simulink model "diff_derive"  (R2019b)
settings: Solver=VariableStepAuto  StartTime=0.0  StopTime=20  RelTol=1e-3
undefined symbols (not defined in the file): d1, DiscIntNeverNeededParam, Goal, p1, p2
libraries: simulink x2
settings Model: Creator=alilf  LastModifiedBy=alilf

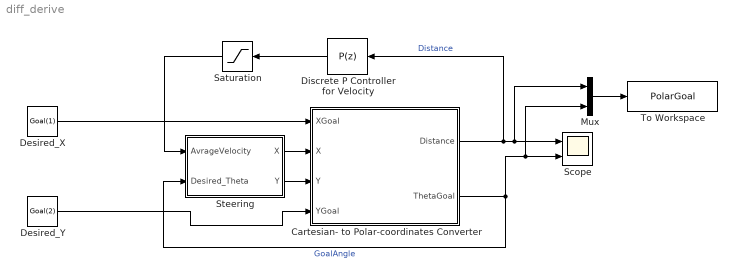
== system diff_derive ==
  "Cartesian- to Polar-coordinates Converter " : MATLAB Function  TreatAsAtomicUnit=on
  Desired_X : Constant  Value=Goal(1)  SampleTime=0.1
  Desired_Y : Constant  Value=Goal(2)  SampleTime=0.1
  Discrete P Controller for Velocity : simulink/Continuous/PID Controller  Controller=P  Form=Parallel  TimeDomain=Discrete-time  SampleTime=0.1  IntegratorMethod=Forward Euler  FilterMethod=Forward Euler  ControllerParametersSource=internal  P=p2  I=1  D=0  UseFilter=on  N=100  TunerSelectOption=Transfer Function Based (PID Tuner App)  InitialConditionSource=internal  InitialConditionForIntegrator=0  InitialConditionForFilter=0  DifferentiatorICPrevScaledInput=0  ExternalReset=none  TrackingMode=off  Kt=1  LimitOutput=off  UpperSaturationLimit=inf  LowerSaturationLimit=-inf  LinearizeAsGain=off  AntiWindupMode=none  Kb=1  POutMin=[]  POutMax=[]  IOutMin=[]  IOutMax=[]  DOutMin=[]  DOutMax=[]  NOutMin=[]  NOutMax=[]  SumOutMin=[]  SumOutMax=[]  SaturationOutMin=[]  SaturationOutMax=[]  PParamMin=[]  PParamMax=[]  IParamMin=[]  IParamMax=[]  DParamMin=[]  DParamMax=[]  NParamMin=[]  NParamMax=[]  KbParamMin=[]  KbParamMax=[]  KtParamMin=[]  KtParamMax=[]  KbOutMin=[]  KbOutMax=[]  KtOutMin=[]  KtOutMax=[]  IntegratorOutMin=[]  IntegratorOutMax=[]  FilterOutMin=[]  FilterOutMax=[]  SumI1OutMin=[]  SumI1OutMax=[]  SumI2OutMin=[]  SumI2OutMax=[]  SumI3OutMin=[]  SumI3OutMax=[]  SumI4OutMin=[]  SumI4OutMax=[]  SumDOutMin=[]  SumDOutMax=[]  DifferentiatorOutMin=[]  DifferentiatorOutMax=[]  FilterDiffOutCoefMin=[]  FilterDiffOutCoefMax=[]  ReciprocalOutMin=[]  ReciprocalOutMax=[]  SumDenOutMin=[]  SumDenOutMax=[]  SumNumOutMin=[]  SumNumOutMax=[]  DivideOutMin=[]  DivideOutMax=[]  IntegratorContinuousStateAttributes=''  IntegratorStateMustResolveToSignalObject=off  IntegratorRTWStateStorageClass=Auto  FilterContinuousStateAttributes=''  FilterStateMustResolveToSignalObject=off  FilterRTWStateStorageClass=Auto  ParallelPVariant=InternalParameters  IdealPVariant=Disabled  IVariant=Disabled  DVariant=Disabled  IntegratorVariant=Disabled  SatVariant=Disabled  AWVariant=Disabled  PCopyVariant=Disabled  TRVariant=Disabled  FdbkBlocksVariant=Forward  IdealPFdbkVariant=Disabled  SatFdbkVariant=Disabled  DerivativeFilterVariant=Disabled  NVariant=Disabled  NCopyVariant=Disabled_SignalSpec  FilterICVariant=Disabled  IntegratorICVariant=Disabled  ExternalResetVariant=Disabled  TRSumVariant=Passthrough  SumFdbkVariant=Disabled  SumVariant=Passthrough_P
  Mux : Mux  Inputs=2
  Saturation : Saturate  UpperLimit=8  LowerLimit=-8
  Scope : Scope  NumInputPorts=2
  "Steering " : Subsystem
  To Workspace : ToWorkspace  VariableName=PolarGoal  SaveFormat=Timeseries  SampleTime=-1
  wires:
  Saturation/1 -> "Steering "/1(AvrageVelocity)
  "Cartesian- to Polar-coordinates Converter "/2(ThetaGoal) -> Mux/2, Scope/2, "Steering "/2(Desired_Theta)  "GoalAngle"
  Discrete P Controller for Velocity/1 -> Saturation/1
  "Cartesian- to Polar-coordinates Converter "/1(Distance) -> Mux/1, Scope/1, Discrete P Controller for Velocity/1  "Distance"
  "Steering "/1(X) -> "Cartesian- to Polar-coordinates Converter "/2(X)
  "Steering "/2(Y) -> "Cartesian- to Polar-coordinates Converter "/3(Y)
  Desired_X/1 -> "Cartesian- to Polar-coordinates Converter "/1(XGoal)
  Desired_Y/1 -> "Cartesian- to Polar-coordinates Converter "/4(YGoal)
  Mux/1 -> To Workspace/1

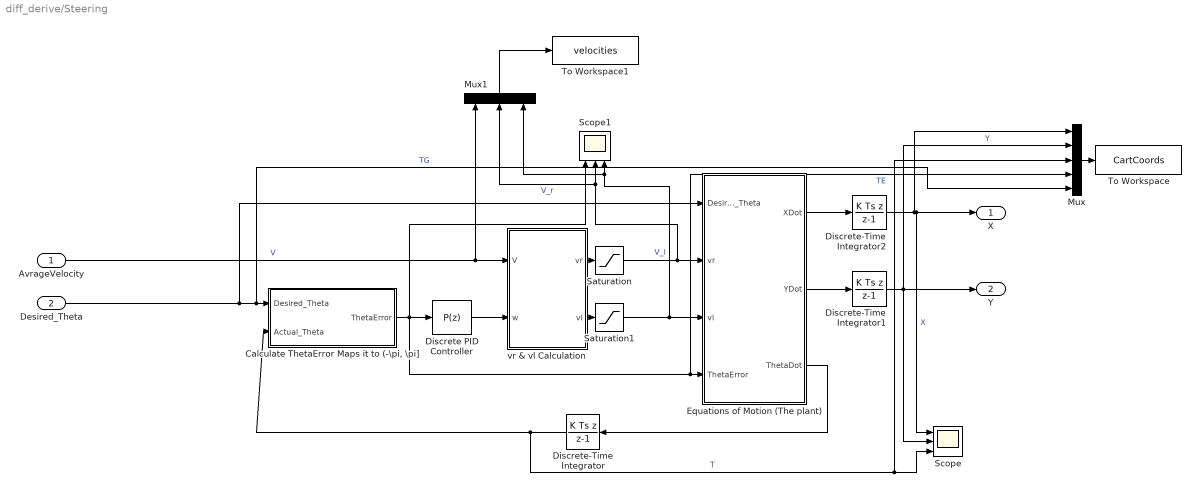
== system diff_derive/Steering  ==
  AvrageVelocity : Inport
  Desired_Theta : Inport  Port=2
  "Calculate ThetaError Maps it to (-\\pi, \\pi]" : MATLAB Function  TreatAsAtomicUnit=on
  Discrete PID Controller : simulink/Continuous/PID Controller  Controller=P  Form=Parallel  TimeDomain=Discrete-time  SampleTime=0.1  IntegratorMethod=Forward Euler  FilterMethod=Forward Euler  ControllerParametersSource=internal  P=p1  I=1  D=d1  UseFilter=on  N=100  TunerSelectOption=Transfer Function Based (PID Tuner App)  InitialConditionSource=internal  InitialConditionForIntegrator=0  InitialConditionForFilter=0  DifferentiatorICPrevScaledInput=0  ExternalReset=none  TrackingMode=off  Kt=1  LimitOutput=off  UpperSaturationLimit=inf  LowerSaturationLimit=-inf  LinearizeAsGain=off  AntiWindupMode=none  Kb=1  POutMin=[]  POutMax=[]  IOutMin=[]  IOutMax=[]  DOutMin=[]  DOutMax=[]  NOutMin=[]  NOutMax=[]  SumOutMin=[]  SumOutMax=[]  SaturationOutMin=[]  SaturationOutMax=[]  PParamMin=[]  PParamMax=[]  IParamMin=[]  IParamMax=[]  DParamMin=[]  DParamMax=[]  NParamMin=[]  NParamMax=[]  KbParamMin=[]  KbParamMax=[]  KtParamMin=[]  KtParamMax=[]  KbOutMin=[]  KbOutMax=[]  KtOutMin=[]  KtOutMax=[]  IntegratorOutMin=[]  IntegratorOutMax=[]  FilterOutMin=[]  FilterOutMax=[]  SumI1OutMin=[]  SumI1OutMax=[]  SumI2OutMin=[]  SumI2OutMax=[]  SumI3OutMin=[]  SumI3OutMax=[]  SumI4OutMin=[]  SumI4OutMax=[]  SumDOutMin=[]  SumDOutMax=[]  DifferentiatorOutMin=[]  DifferentiatorOutMax=[]  FilterDiffOutCoefMin=[]  FilterDiffOutCoefMax=[]  ReciprocalOutMin=[]  ReciprocalOutMax=[]  SumDenOutMin=[]  SumDenOutMax=[]  SumNumOutMin=[]  SumNumOutMax=[]  DivideOutMin=[]  DivideOutMax=[]  IntegratorContinuousStateAttributes=''  IntegratorStateMustResolveToSignalObject=off  IntegratorRTWStateStorageClass=Auto  FilterContinuousStateAttributes=''  FilterStateMustResolveToSignalObject=off  FilterRTWStateStorageClass=Auto  ParallelPVariant=InternalParameters  IdealPVariant=Disabled  IVariant=Disabled  DVariant=Disabled  IntegratorVariant=Disabled  SatVariant=Disabled  AWVariant=Disabled  PCopyVariant=Disabled  TRVariant=Disabled  FdbkBlocksVariant=Forward  IdealPFdbkVariant=Disabled  SatFdbkVariant=Disabled  DerivativeFilterVariant=Disabled  NVariant=Disabled  NCopyVariant=Disabled_SignalSpec  FilterICVariant=Disabled  IntegratorICVariant=Disabled  ExternalResetVariant=Disabled  TRSumVariant=Passthrough  SumFdbkVariant=Disabled  SumVariant=Passthrough_P
  Discrete-Time Integrator : DiscreteIntegrator  IntegratorMethod=Integration: Backward Euler  SampleTime=0.1  ICPrevOutput=DiscIntNeverNeededParam  ICPrevScaledInput=DiscIntNeverNeededParam
  Discrete-Time Integrator1 : DiscreteIntegrator  IntegratorMethod=Integration: Backward Euler  SampleTime=0.1  ICPrevOutput=DiscIntNeverNeededParam  ICPrevScaledInput=DiscIntNeverNeededParam
  Discrete-Time Integrator2 : DiscreteIntegrator  IntegratorMethod=Integration: Backward Euler  SampleTime=0.1  ICPrevOutput=DiscIntNeverNeededParam  ICPrevScaledInput=DiscIntNeverNeededParam
  Equations of Motion (The plant) : MATLAB Function  TreatAsAtomicUnit=on  SystemSampleTime=0.1
  Mux : Mux  Inputs=5
  Mux1 : Mux  Inputs=3
  Saturation : Saturate  UpperLimit=10  LowerLimit=-10
  Saturation1 : Saturate  UpperLimit=10  LowerLimit=-10
  Scope : Scope  NumInputPorts=3
  Scope1 : Scope  NumInputPorts=3
  To Workspace : ToWorkspace  VariableName=CartCoords  SaveFormat=Timeseries  SampleTime=-1
  To Workspace1 : ToWorkspace  VariableName=velocities  SaveFormat=Timeseries  SampleTime=-1
  vr & vl Calculation : MATLAB Function  TreatAsAtomicUnit=on  SystemSampleTime=0.1
  X : Outport
  Y : Outport  Port=2
  wires:
  vr & vl Calculation/1(vr) -> Saturation/1
  Discrete-Time Integrator2/1 -> Mux/1, X/1, Scope/1  "X"
  Discrete PID Controller/1 -> vr & vl Calculation/2(w)
  Equations of Motion (The plant)/1(XDot) -> Discrete-Time Integrator2/1
  Desired_Theta/1 -> Mux/5, "Calculate ThetaError Maps it to (-\\pi, \\pi]"/1(Desired_Theta), Equations of Motion (The plant)/1(Desired_Theta)  "TG"
  "Calculate ThetaError Maps it to (-\\pi, \\pi]"/1(ThetaError) -> Mux/4, Equations of Motion (The plant)/4(ThetaError), Discrete PID Controller/1, Scope1/1  "TE"
  Equations of Motion (The plant)/3(ThetaDot) -> Discrete-Time Integrator/1
  Saturation1/1 -> Equations of Motion (The plant)/3(vl), Mux1/3, Scope1/3  "V_l"
  Discrete-Time Integrator/1 -> "Calculate ThetaError Maps it to (-\\pi, \\pi]"/2(Actual_Theta), Mux/3, Scope/3  "T"
  Saturation/1 -> Mux1/2, Scope1/2, Equations of Motion (The plant)/2(vr)  "V_r"
  vr & vl Calculation/2(vl) -> Saturation1/1
  Discrete-Time Integrator1/1 -> Mux/2, Y/1, Scope/2  "Y"
  AvrageVelocity/1 -> vr & vl Calculation/1(V), Mux1/1  "V"
  Equations of Motion (The plant)/2(YDot) -> Discrete-Time Integrator1/1
  Mux/1 -> To Workspace/1
  Mux1/1 -> To Workspace1/1

== matlab function diff_derive/Steering /Equations of Motion (The plant) ==
  data: Desired_Theta input; vr input; XDot output; vl input; YDot output; ThetaDot output; ThetaError input
function [XDot, YDot, ThetaDot] = fcn(Desired_Theta, vr, vl, ThetaError )
L = 21; %the width of the robot in [cm]
Theta = Desired_Theta - ThetaError;
V = vr + vl;
XDot = V * cos(Theta) / 2;
YDot = V * sin(Theta) / 2;
ThetaDot = (vr - vl) / L;

== matlab function diff_derive/Steering /vr & vl Calculation ==
  data: V input; vr output; w input; vl output
function [vr, vl] = fcn(V,w)
L = 21; %the width of the robot in [cm]
vr = V + L*w/2;
vl = V - L*w/2;

== matlab function diff_derive/Steering /Calculate ThetaError Maps it to (-\pi, \pi] ==
  data: Desired_Theta input; ThetaError output; Actual_Theta input
function ThetaError = fcn(Desired_Theta, Actual_Theta)
%Calculate ThetaError
%Maps it to (-\pi, \pi]

TDiff = (Desired_Theta - Actual_Theta);
ThetaError = atan2(sin(TDiff), cos(TDiff));

== matlab function diff_derive/Cartesian- to Polar-coordinates Converter  ==
  data: XGoal input; Distance output; X input; Y input; YGoal input; ThetaGoal output
function [Distance, ThetaGoal] = fcn(XGoal, X, Y, YGoal)
x = XGoal - X;
y = YGoal - Y;
Distance = sqrt(x^2 + y^2);
ThetaGoal = atan2(y, x);
